simulink library "AERO_lib"  (R2015a)
settings: Solver=ode45  StartTime=0.0  StopTime=10.0  RelTol=1e-3
values from neighbouring files (symbols this model uses):
  AERO = AEROmod    [setup_aero.m]
undefined symbols (not defined in the file or in its folder): VAF
libraries: STRUCT_MDL x2, simulink x2
settings Model: Creator=Andrew  LastModifiedBy=Andrew

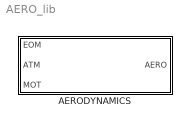
== system AERO_lib ==
  AERODYNAMICS : Subsystem

== system AERO_lib/AERODYNAMICS ==
  EOM : Inport
  ATM : Inport  Port=2
  MOT : Inport  Port=3
  AERODYNAMICS : Subsystem
  Bus Creator : BusCreator  Inputs=3
  Bus Selector : BusSelector  OutputSignals=SONIC_VEL,TEMP,RHO
  Bus Selector1 : BusSelector  OutputSignals=signal1,signal2
  Bus Selector2 : BusSelector  OutputSignals=signal1,signal2
  AERO : Outport
  wires:
  Bus Selector2/2 -> AERODYNAMICS/9(MOTOR DIAMETER)  "<signal2>"
  Bus Selector2/1 -> AERODYNAMICS/8(THRUST ACTIVE)  "<signal1>"
  Bus Selector/3 -> AERODYNAMICS/7(RHO)  "<RHO>"
  Bus Selector/2 -> AERODYNAMICS/6(TEMP)  "<TEMP>"
  Bus Selector/1 -> AERODYNAMICS/5(a (m/s))  "<SONIC_VEL>"
  Bus Creator/1 -> AERO/1
  ATM/1 -> Bus Selector/1
  EOM/1 -> Bus Selector1/1
  MOT/1 -> Bus Selector2/1
  AERODYNAMICS/2(VEHICLE) -> Bus Creator/2  "VEHICLE"
  AERODYNAMICS/3(FLUID) -> Bus Creator/3  "FLUID"
  AERODYNAMICS/1(AERO_PROP) -> Bus Creator/1  "AERO_PROP"

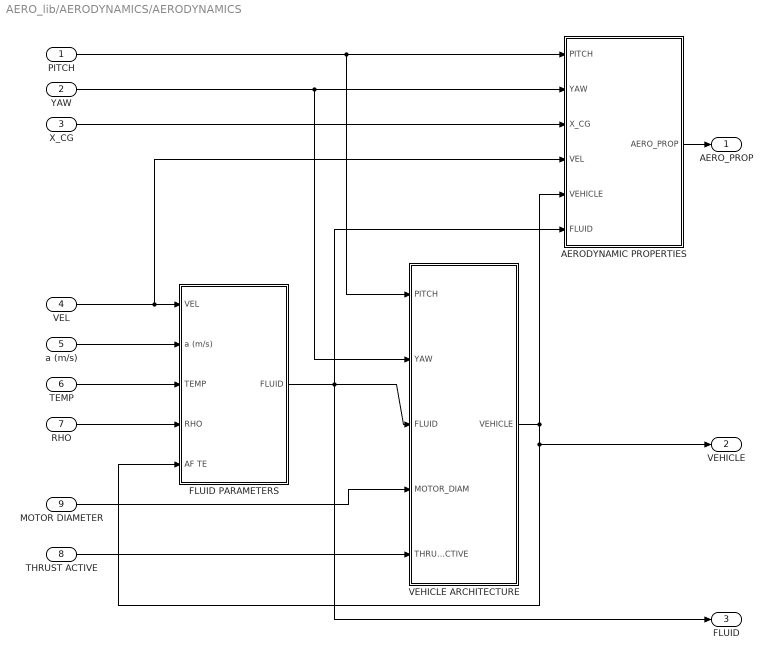
== system AERO_lib/AERODYNAMICS/AERODYNAMICS ==
  PITCH : Inport
  YAW : Inport  Port=2
  X_CG : Inport  Port=3
  VEL : Inport  Port=4
  a (m/s) : Inport  Port=5
  TEMP : Inport  Port=6
  RHO : Inport  Port=7
  THRUST ACTIVE : Inport  Port=8
  MOTOR DIAMETER : Inport  Port=9
  AERODYNAMIC PROPERTIES : Subsystem
  FLUID PARAMETERS : Subsystem
  VEHICLE ARCHITECTURE : Subsystem
  AERO_PROP : Outport
  VEHICLE : Outport  Port=2
  FLUID : Outport  Port=3
  wires:
  TEMP/1 -> FLUID PARAMETERS/3(TEMP)
  THRUST ACTIVE/1 -> VEHICLE ARCHITECTURE/5(THRUST_ACTIVE)
  MOTOR DIAMETER/1 -> VEHICLE ARCHITECTURE/4(MOTOR_DIAM)
  VEHICLE ARCHITECTURE/1(VEHICLE) -> FLUID PARAMETERS/5(AF TE), VEHICLE/1, AERODYNAMIC PROPERTIES/5(VEHICLE)
  RHO/1 -> FLUID PARAMETERS/4(RHO)
  a (m/s)/1 -> FLUID PARAMETERS/2(a (m/s))
  PITCH/1 -> VEHICLE ARCHITECTURE/1(PITCH), AERODYNAMIC PROPERTIES/1(PITCH)
  VEL/1 -> AERODYNAMIC PROPERTIES/4(VEL), FLUID PARAMETERS/1(VEL)
  X_CG/1 -> AERODYNAMIC PROPERTIES/3(X_CG)
  FLUID PARAMETERS/1(FLUID) -> AERODYNAMIC PROPERTIES/6(FLUID), VEHICLE ARCHITECTURE/3(FLUID), FLUID/1
  AERODYNAMIC PROPERTIES/1(AERO_PROP) -> AERO_PROP/1
  YAW/1 -> VEHICLE ARCHITECTURE/2(YAW), AERODYNAMIC PROPERTIES/2(YAW)

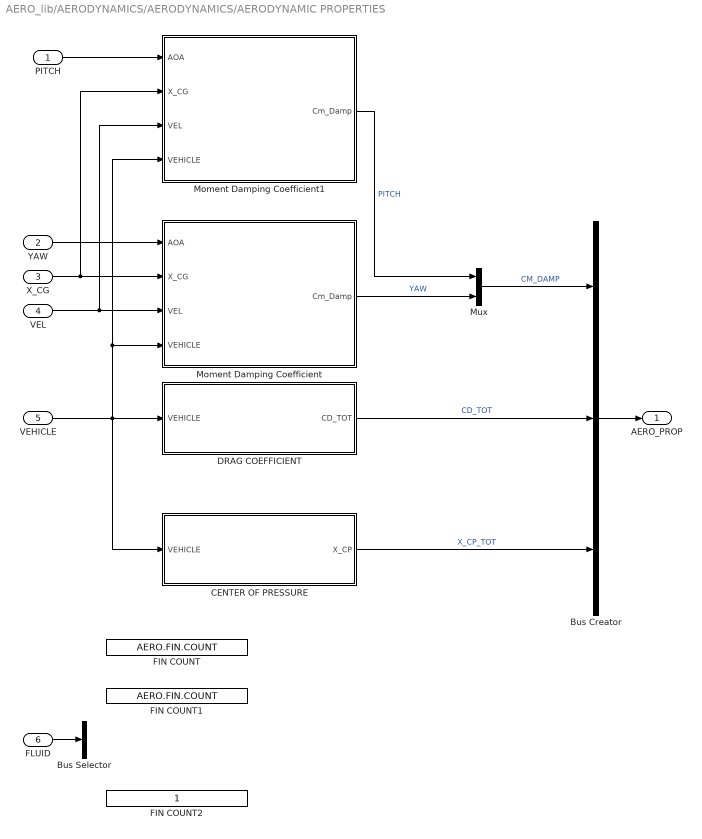
== system AERO_lib/AERODYNAMICS/AERODYNAMICS/AERODYNAMIC PROPERTIES ==
  PITCH : Inport
  YAW : Inport  Port=2
  X_CG : Inport  Port=3
  VEL : Inport  Port=4
  VEHICLE : Inport  Port=5
  FLUID : Inport  Port=6
  Bus Creator : BusCreator  Inputs=3
  Bus Selector : BusSelector  OutputSignals=MACH
  CENTER OF PRESSURE : Subsystem
  DRAG COEFFICIENT : Subsystem
  FIN COUNT : Constant  Value=AERO.FIN.COUNT
  FIN COUNT1 : Constant  Value=AERO.FIN.COUNT
  FIN COUNT2 : Constant
  Moment Damping Coefficient : Subsystem
  Moment Damping Coefficient1 : Subsystem
  Mux : Mux  Inputs=2
  AERO_PROP : Outport
  wires:
  VEL/1 -> Moment Damping Coefficient/3(VEL), Moment Damping Coefficient1/3(VEL)
  X_CG/1 -> Moment Damping Coefficient/2(X_CG), Moment Damping Coefficient1/2(X_CG)
  PITCH/1 -> Moment Damping Coefficient1/1(AOA)
  VEHICLE/1 -> CENTER OF PRESSURE/1(VEHICLE), Moment Damping Coefficient1/4(VEHICLE), Moment Damping Coefficient/4(VEHICLE), DRAG COEFFICIENT/1(VEHICLE)
  DRAG COEFFICIENT/1(CD_TOT) -> Bus Creator/2  "CD_TOT"
  CENTER OF PRESSURE/1(X_CP) -> Bus Creator/3  "X_CP_TOT"
  Bus Creator/1 -> AERO_PROP/1
  YAW/1 -> Moment Damping Coefficient/1(AOA)
  Moment Damping Coefficient/1(Cm_Damp) -> Mux/2  "YAW"
  Moment Damping Coefficient1/1(Cm_Damp) -> Mux/1  "PITCH"
  Mux/1 -> Bus Creator/1  "CM_DAMP"
  FLUID/1 -> Bus Selector/1

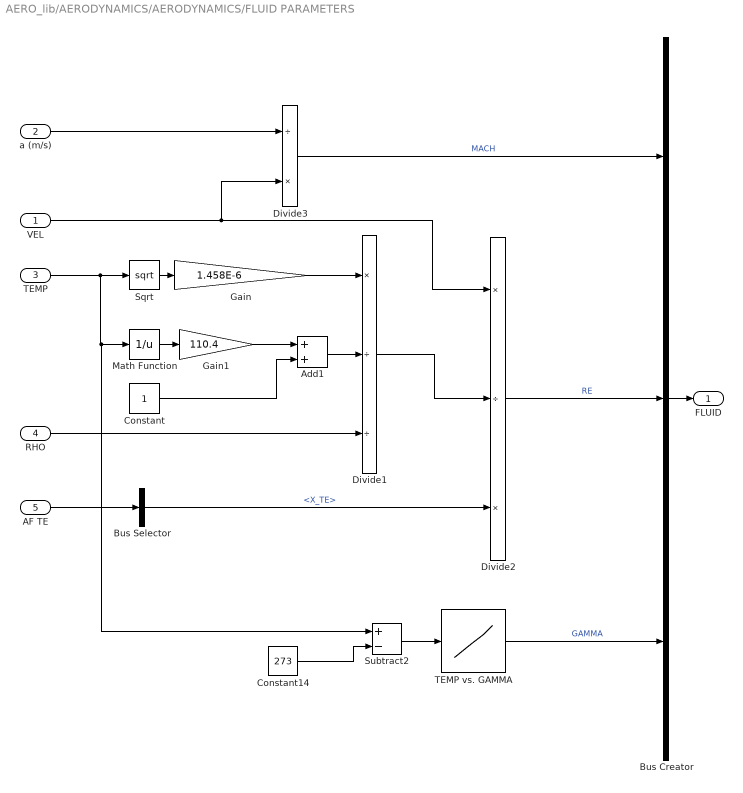
== system AERO_lib/AERODYNAMICS/AERODYNAMICS/FLUID PARAMETERS ==
  VEL : Inport
  a (m/s) : Inport  Port=2
  TEMP : Inport  Port=3
  RHO : Inport  Port=4
  AF TE : Inport  Port=5
  Add1 : Sum
  Bus Creator : BusCreator  Inputs=3
  Bus Selector : BusSelector  OutputSignals=AIRFRAME.AF_2.X_TE
  Constant : Constant
  Constant14 : Constant  Value=273
  Divide1 : Product  Inputs=*//
  Divide2 : Product  Inputs=*/*
  Divide3 : Product  Inputs=/*
  Gain : Gain  Gain=1.458E-6
  Gain1 : Gain  Gain=110.4
  Math Function : Math  Operator=reciprocal  SaturateOnIntegerOverflow=on
  Sqrt : Sqrt  SaturateOnIntegerOverflow=on
  Subtract2 : Sum  Inputs=+-
  TEMP vs. GAMMA : Lookup_n-D  NumberOfTableDimensions=1  BreakpointsForDimension1=VAF.GAS.GAMMA_VS_TEMP(:,1)  Table=VAF.GAS.GAMMA_VS_TEMP(:,2)  InternalRulePriority=Speed  RndMeth=Simplest  InputSameDT=on
  FLUID : Outport
  wires:
  Constant/1 -> Add1/2
  Math Function/1 -> Gain1/1
  Gain1/1 -> Add1/1
  RHO/1 -> Divide1/3
  Add1/1 -> Divide1/2
  Divide1/1 -> Divide2/2
  Sqrt/1 -> Gain/1
  Gain/1 -> Divide1/1
  Divide2/1 -> Bus Creator/2  "RE"
  VEL/1 -> Divide3/2, Divide2/1
  a (m/s)/1 -> Divide3/1
  Divide3/1 -> Bus Creator/1  "MACH"
  Subtract2/1 -> TEMP vs. GAMMA/1
  TEMP/1 -> Subtract2/1, Math Function/1, Sqrt/1
  Constant14/1 -> Subtract2/2
  TEMP vs. GAMMA/1 -> Bus Creator/3  "GAMMA"
  AF TE/1 -> Bus Selector/1
  Bus Selector/1 -> Divide2/3  "<X_TE>"
  Bus Creator/1 -> FLUID/1

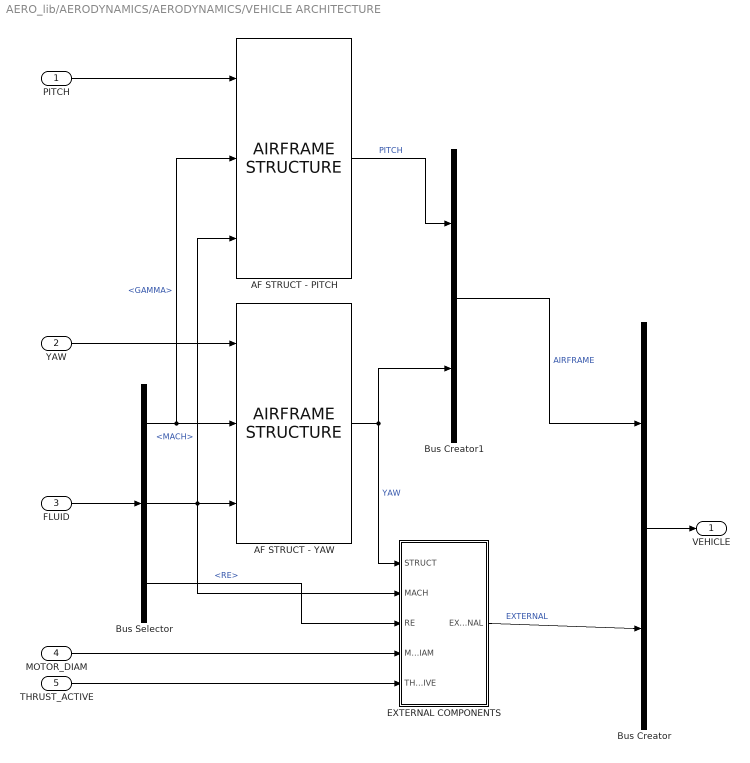
== system AERO_lib/AERODYNAMICS/AERODYNAMICS/VEHICLE ARCHITECTURE ==
  PITCH : Inport
  YAW : Inport  Port=2
  FLUID : Inport  Port=3
  MOTOR_DIAM : Inport  Port=4
  THRUST_ACTIVE : Inport  Port=5
  AF STRUCT - PITCH : STRUCT_MDL/AIRFRAME STRUCTURE
  AF STRUCT - YAW : STRUCT_MDL/AIRFRAME STRUCTURE
  Bus Creator : BusCreator  Inputs=2
  Bus Creator1 : BusCreator  Inputs=2
  Bus Selector : BusSelector  OutputSignals=GAMMA,MACH,RE
  EXTERNAL COMPONENTS : Subsystem
  VEHICLE : Outport
  wires:
  MOTOR_DIAM/1 -> EXTERNAL COMPONENTS/4(MOTOR_DIAM)
  THRUST_ACTIVE/1 -> EXTERNAL COMPONENTS/5(THRUST_ACTIVE)
  AF STRUCT - YAW/1 -> EXTERNAL COMPONENTS/1(STRUCT), Bus Creator1/2  "YAW"
  EXTERNAL COMPONENTS/1(EXTERNAL) -> Bus Creator/2  "EXTERNAL"
  Bus Creator/1 -> VEHICLE/1
  FLUID/1 -> Bus Selector/1
  Bus Selector/1 -> AF STRUCT - PITCH/2, AF STRUCT - YAW/2  "<GAMMA>"
  Bus Selector/3 -> EXTERNAL COMPONENTS/3(RE)  "<RE>"
  Bus Selector/2 -> AF STRUCT - PITCH/3, AF STRUCT - YAW/3, EXTERNAL COMPONENTS/2(MACH)  "<MACH>"
  PITCH/1 -> AF STRUCT - PITCH/1
  YAW/1 -> AF STRUCT - YAW/1
  Bus Creator1/1 -> Bus Creator/1  "AIRFRAME"
  AF STRUCT - PITCH/1 -> Bus Creator1/1  "PITCH"

== system AERO_lib/AERODYNAMICS/AERODYNAMICS/AERODYNAMIC PROPERTIES/CENTER OF PRESSURE ==
  VEHICLE : Inport
  Bus Selector : BusSelector  OutputSignals=NC.CP,AF_1.CP,AF_2.CP,FIN.CP,NC.CN_ALPHA,AF_1.CN_ALPHA,AF_2.CN_ALPHA,FIN.CN_ALPHA
  Divide : Product  Inputs=*/
  Dot Product : DotProduct  InputSameDT=on  OutDataTypeStr=Inherit: Inherit via internal rule
  Mux : Mux
  Mux1 : Mux
  Sum of Elements1 : Sum  Inputs=+
  X_CP : Outport
  wires:
  Divide/1 -> X_CP/1  "X_CP_TOT"
  VEHICLE/1 -> Bus Selector/1
  Mux1/1 -> Dot Product/2, Sum of Elements1/1
  Sum of Elements1/1 -> Divide/2
  Mux/1 -> Dot Product/1
  Bus Selector/4 -> Mux/4  "<CP>"
  Bus Selector/3 -> Mux/3  "<CP>"
  Bus Selector/2 -> Mux/2  "<CP>"
  Bus Selector/1 -> Mux/1  "<CP>"
  Bus Selector/5 -> Mux1/1  "<CN_ALPHA>"
  Bus Selector/6 -> Mux1/2  "<CN_ALPHA>"
  Bus Selector/7 -> Mux1/3  "<CN_ALPHA>"
  Bus Selector/8 -> Mux1/4  "<CN_ALPHA>"
  Dot Product/1 -> Divide/1

== system AERO_lib/AERODYNAMICS/AERODYNAMICS/AERODYNAMIC PROPERTIES/DRAG COEFFICIENT ==
  VEHICLE : Inport
  Add1 : Sum
  Bus Selector1 : BusSelector  OutputSignals=EXTERNAL.SKIN_EFFECTS,AIRFRAME.NC.CD,AIRFRAME.FIN.CD,EXTERNAL.BASE.CD_BASE,EXTERNAL.PARASITIC.CD_PARASITIC,AIRFRAME.NC.REF_AREA,AIRFRAME.FIN.REF_AREA,EXTERNAL.BASE.BASE_REF_AREA,EXTERNAL.PARASITIC.AREA_PARASITIC,AIRFRAME.AF_1.AREA_LE
  Divide1 : Product  Inputs=*/
  Dot Product1 : DotProduct  InputSameDT=on  OutDataTypeStr=Inherit: Inherit via internal rule
  Mux3 : Mux
  Mux4 : Mux
  CD_TOT : Outport
  wires:
  Mux3/1 -> Dot Product1/1
  VEHICLE/1 -> Bus Selector1/1
  Mux4/1 -> Dot Product1/2
  Dot Product1/1 -> Divide1/1
  Bus Selector1/7 -> Mux4/2  "<REF_AREA>"
  Bus Selector1/8 -> Mux4/3  "<BASE_REF_AREA>"
  Bus Selector1/9 -> Mux4/4  "<AREA_PARASITIC>"
  Bus Selector1/2 -> Mux3/1  "<CD>"
  Bus Selector1/1 -> Add1/1  "<SKIN_EFFECTS>"
  Divide1/1 -> Add1/2
  Add1/1 -> CD_TOT/1  "CD_TOT"
  Bus Selector1/6 -> Mux4/1  "<REF_AREA>"
  Bus Selector1/4 -> Mux3/3  "<CD_BASE>"
  Bus Selector1/3 -> Mux3/2  "<CD>"
  Bus Selector1/5 -> Mux3/4  "<CD_PARASITIC>"
  Bus Selector1/10 -> Divide1/2  "<AREA_LE>"

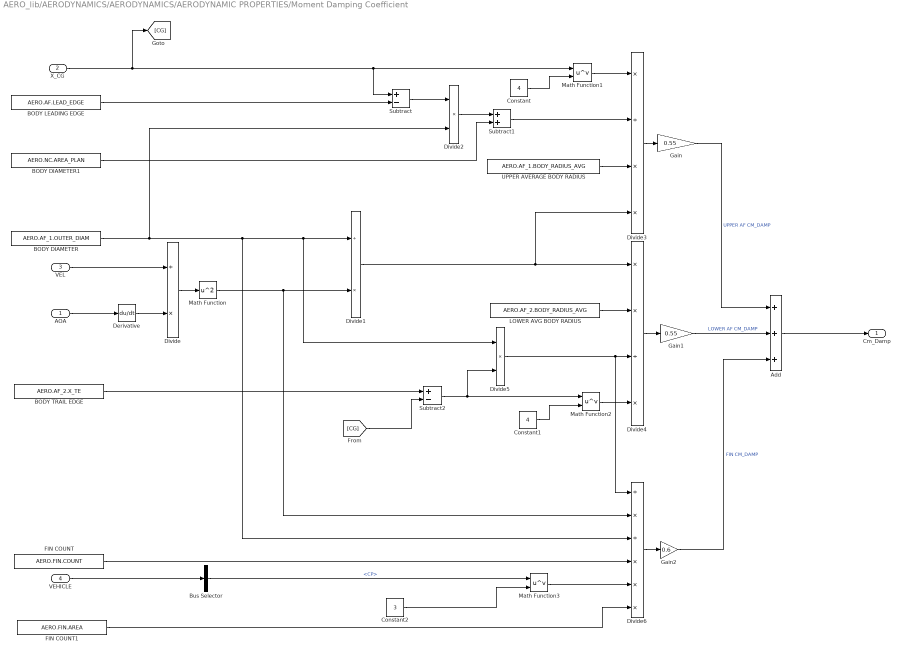
== system AERO_lib/AERODYNAMICS/AERODYNAMICS/AERODYNAMIC PROPERTIES/Moment Damping Coefficient ==
  AOA : Inport
  X_CG : Inport  Port=2
  VEL : Inport  Port=3
  VEHICLE : Inport  Port=4
  Add : Sum  Inputs=+++
  BODY DIAMETER : FromWorkspace  VariableName=AERO.AF_1.OUTER_DIAM  SampleTime=0
  BODY DIAMETER1 : FromWorkspace  VariableName=AERO.NC.AREA_PLAN  SampleTime=0
  BODY LEADING EDGE : FromWorkspace  VariableName=AERO.AF.LEAD_EDGE  SampleTime=0
  BODY TRAIL EDGE : Constant  Value=AERO.AF_2.X_TE
  Bus Selector : BusSelector  OutputSignals=AIRFRAME.YAW.FIN.CP
  Constant : Constant  Value=4
  Constant1 : Constant  Value=4
  Constant2 : Constant  Value=3
  Derivative : Derivative
  Divide : Product  Inputs=/*
  Divide1 : Product  Inputs=/*
  Divide2 : Product  Inputs=**
  Divide3 : Product  Inputs=*/**
  Divide4 : Product  Inputs=**/*
  Divide5 : Product  Inputs=**
  Divide6 : Product  Inputs=/*/***
  FIN COUNT : Constant  Value=AERO.FIN.COUNT
  FIN COUNT1 : FromWorkspace  VariableName=AERO.FIN.AREA  SampleTime=0
  Gain : Gain  Gain=0.55
  Gain1 : Gain  Gain=0.55
  Gain2 : Gain  Gain=0.6
  LOWER AVG BODY RADIUS : FromWorkspace  VariableName=AERO.AF_2.BODY_RADIUS_AVG  SampleTime=0
  Math Function : Math  Operator=square  SaturateOnIntegerOverflow=on
  Math Function1 : Math  Operator=pow  SaturateOnIntegerOverflow=on
  Math Function2 : Math  Operator=pow  SaturateOnIntegerOverflow=on
  Math Function3 : Math  Operator=pow  SaturateOnIntegerOverflow=on
  Subtract : Sum  Inputs=+-
  Subtract1 : Sum
  Subtract2 : Sum  Inputs=+-
  UPPER AVERAGE BODY RADIUS : Constant  Value=AERO.AF_1.BODY_RADIUS_AVG
  Cm_Damp : Outport
  wires:
  Derivative/1 -> Divide/2
  VEL/1 -> Divide/1
  Divide/1 -> Math Function/1
  Math Function/1 -> Divide6/2, Divide1/2
  BODY LEADING EDGE/1 -> Subtract/2
  Divide2/1 -> Subtract1/1
  Constant/1 -> Math Function1/2
  Subtract/1 -> Divide2/1
  Subtract1/1 -> Divide3/2
  BODY DIAMETER1/1 -> Subtract1/2
  BODY DIAMETER/1 -> Divide6/3, Divide5/1, Divide1/1, Divide2/2
  X_CG/1 -> [CG], Subtract/1, Math Function1/1
  Math Function1/1 -> Divide3/1
  Divide3/1 -> Gain/1
  BODY TRAIL EDGE/1 -> Subtract2/1
  [CG] -> Subtract2/2
  Divide5/1 -> Divide6/1, Divide4/3
  Subtract2/1 -> Math Function2/1, Divide5/2
  Constant1/1 -> Math Function2/2
  Divide4/1 -> Gain1/1
  VEHICLE/1 -> Bus Selector/1
  Constant2/1 -> Math Function3/2
  Math Function3/1 -> Divide6/5
  FIN COUNT/1 -> Divide6/4
  FIN COUNT1/1 -> Divide6/6
  Divide6/1 -> Gain2/1
  Gain1/1 -> Add/2  "LOWER AF CM_DAMP"
  Gain2/1 -> Add/3  "FIN CM_DAMP"
  Gain/1 -> Add/1  "UPPER AF CM_DAMP"
  UPPER AVERAGE BODY RADIUS/1 -> Divide3/3
  Divide1/1 -> Divide3/4, Divide4/1
  Math Function2/1 -> Divide4/4
  LOWER AVG BODY RADIUS/1 -> Divide4/2
  Bus Selector/1 -> Math Function3/1  "<CP>"
  AOA/1 -> Derivative/1
  Add/1 -> Cm_Damp/1

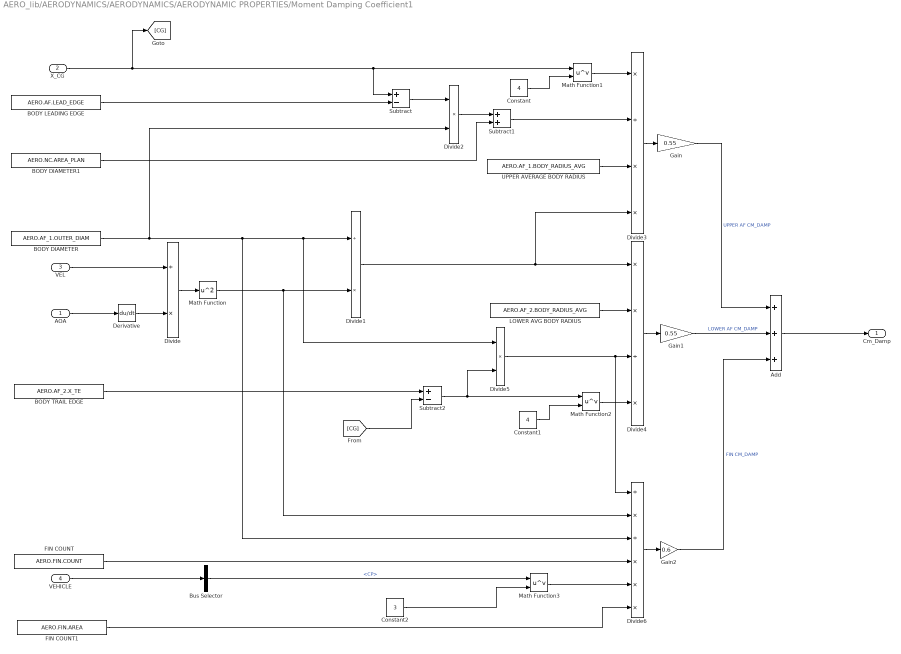
== system AERO_lib/AERODYNAMICS/AERODYNAMICS/AERODYNAMIC PROPERTIES/Moment Damping Coefficient1 ==
  AOA : Inport
  X_CG : Inport  Port=2
  VEL : Inport  Port=3
  VEHICLE : Inport  Port=4
  Add : Sum  Inputs=+++
  BODY DIAMETER : FromWorkspace  VariableName=AERO.AF_1.OUTER_DIAM  SampleTime=0
  BODY DIAMETER1 : FromWorkspace  VariableName=AERO.NC.AREA_PLAN  SampleTime=0
  BODY LEADING EDGE : FromWorkspace  VariableName=AERO.AF.LEAD_EDGE  SampleTime=0
  BODY TRAIL EDGE : Constant  Value=AERO.AF_2.X_TE
  Bus Selector : BusSelector  OutputSignals=AIRFRAME.PITCH.FIN.CP
  Constant : Constant  Value=4
  Constant1 : Constant  Value=4
  Constant2 : Constant  Value=3
  Derivative : Derivative
  Divide : Product  Inputs=/*
  Divide1 : Product  Inputs=/*
  Divide2 : Product  Inputs=**
  Divide3 : Product  Inputs=*/**
  Divide4 : Product  Inputs=**/*
  Divide5 : Product  Inputs=**
  Divide6 : Product  Inputs=/*/***
  FIN COUNT : Constant  Value=AERO.FIN.COUNT
  FIN COUNT1 : FromWorkspace  VariableName=AERO.FIN.AREA  SampleTime=0
  Gain : Gain  Gain=0.55
  Gain1 : Gain  Gain=0.55
  Gain2 : Gain  Gain=0.6
  LOWER AVG BODY RADIUS : FromWorkspace  VariableName=AERO.AF_2.BODY_RADIUS_AVG  SampleTime=0
  Math Function : Math  Operator=square  SaturateOnIntegerOverflow=on
  Math Function1 : Math  Operator=pow  SaturateOnIntegerOverflow=on
  Math Function2 : Math  Operator=pow  SaturateOnIntegerOverflow=on
  Math Function3 : Math  Operator=pow  SaturateOnIntegerOverflow=on
  Subtract : Sum  Inputs=+-
  Subtract1 : Sum
  Subtract2 : Sum  Inputs=+-
  UPPER AVERAGE BODY RADIUS : Constant  Value=AERO.AF_1.BODY_RADIUS_AVG
  Cm_Damp : Outport
  wires:
  Add/1 -> Cm_Damp/1
  AOA/1 -> Derivative/1
  Bus Selector/1 -> Math Function3/1  "<CP>"
  LOWER AVG BODY RADIUS/1 -> Divide4/2
  Math Function2/1 -> Divide4/4
  Divide1/1 -> Divide4/1, Divide3/4
  UPPER AVERAGE BODY RADIUS/1 -> Divide3/3
  Gain/1 -> Add/1  "UPPER AF CM_DAMP"
  Gain2/1 -> Add/3  "FIN CM_DAMP"
  Gain1/1 -> Add/2  "LOWER AF CM_DAMP"
  Divide6/1 -> Gain2/1
  FIN COUNT1/1 -> Divide6/6
  FIN COUNT/1 -> Divide6/4
  Math Function3/1 -> Divide6/5
  Constant2/1 -> Math Function3/2
  VEHICLE/1 -> Bus Selector/1
  Divide4/1 -> Gain1/1
  Constant1/1 -> Math Function2/2
  Subtract2/1 -> Divide5/2, Math Function2/1
  Divide5/1 -> Divide4/3, Divide6/1
  [CG] -> Subtract2/2
  BODY TRAIL EDGE/1 -> Subtract2/1
  Divide3/1 -> Gain/1
  Math Function1/1 -> Divide3/1
  X_CG/1 -> Math Function1/1, Subtract/1, [CG]
  BODY DIAMETER/1 -> Divide2/2, Divide1/1, Divide5/1, Divide6/3
  BODY DIAMETER1/1 -> Subtract1/2
  Subtract1/1 -> Divide3/2
  Subtract/1 -> Divide2/1
  Constant/1 -> Math Function1/2
  Divide2/1 -> Subtract1/1
  BODY LEADING EDGE/1 -> Subtract/2
  Math Function/1 -> Divide1/2, Divide6/2
  Divide/1 -> Math Function/1
  VEL/1 -> Divide/1
  Derivative/1 -> Divide/2

== system AERO_lib/AERODYNAMICS/AERODYNAMICS/VEHICLE ARCHITECTURE/EXTERNAL COMPONENTS ==
  STRUCT : Inport
  MACH : Inport  Port=2
  RE : Inport  Port=3
  MOTOR_DIAM : Inport  Port=4
  THRUST_ACTIVE : Inport  Port=5
  BASE : Subsystem
  Bus Creator : BusCreator  Inputs=3
  Bus Selector : BusSelector  OutputSignals=AF_2.AREA_TE
  PARASITIC : Subsystem
  Skin Friction Drag : Subsystem
  EXTERNAL : Outport
  wires:
  THRUST_ACTIVE/1 -> BASE/3(THRUST ACTIVE)
  MOTOR_DIAM/1 -> BASE/2(MOTOR DIAMETER)
  RE/1 -> Skin Friction Drag/1(Re)
  BASE/1(BASE) -> Bus Creator/1  "BASE"
  Skin Friction Drag/1(Cd_Fric) -> Bus Creator/3  "SKIN_EFFECTS"
  Bus Creator/1 -> EXTERNAL/1
  MACH/1 -> Skin Friction Drag/2(MACH), PARASITIC/1(MACH), BASE/1(MACH)
  STRUCT/1 -> Bus Selector/1
  Bus Selector/1 -> BASE/4(AF TE AREA)  "<AREA_TE>"
  PARASITIC/1(PARASITIC) -> Bus Creator/2  "PARASITIC"

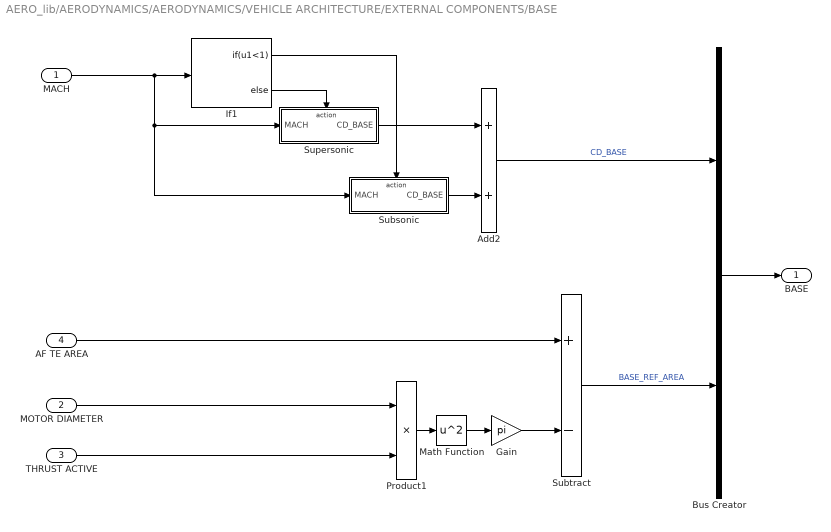
== system AERO_lib/AERODYNAMICS/AERODYNAMICS/VEHICLE ARCHITECTURE/EXTERNAL COMPONENTS/BASE ==
  MACH : Inport
  MOTOR DIAMETER : Inport  Port=2
  THRUST ACTIVE : Inport  Port=3
  AF TE AREA : Inport  Port=4
  Add2 : Sum
  Bus Creator : BusCreator  Inputs=2
  Gain : Gain  Gain=pi
  If1 : If  IfExpression=u1<1
  Math Function : Math  Operator=square  SaturateOnIntegerOverflow=on
  Product1 : Product
  Subsonic : Subsystem  TreatAsAtomicUnit=on
  Subtract : Sum  Inputs=+-
  Supersonic : Subsystem  TreatAsAtomicUnit=on
  BASE : Outport
  wires:
  Add2/1 -> Bus Creator/1  "CD_BASE"
  Subtract/1 -> Bus Creator/2  "BASE_REF_AREA"
  AF TE AREA/1 -> Subtract/1
  Product1/1 -> Math Function/1
  THRUST ACTIVE/1 -> Product1/2
  MOTOR DIAMETER/1 -> Product1/1
  Gain/1 -> Subtract/2
  Math Function/1 -> Gain/1
  If1/2 -> Supersonic/Action
  If1/1 -> Subsonic/Action
  Subsonic/1(CD_BASE) -> Add2/2
  Supersonic/1(CD_BASE) -> Add2/1
  MACH/1 -> Subsonic/1(MACH), Supersonic/1(MACH), If1/1
  Bus Creator/1 -> BASE/1

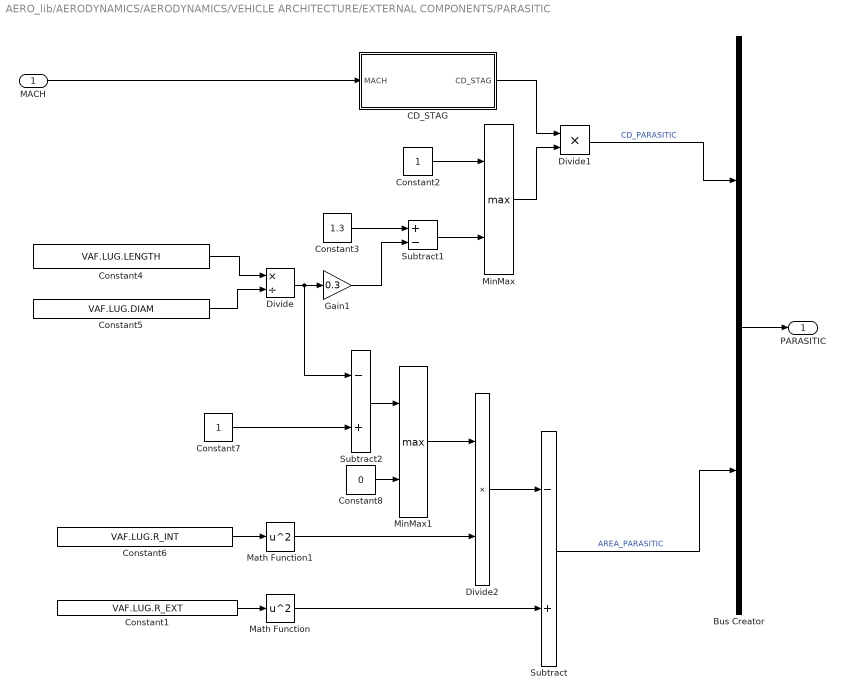
== system AERO_lib/AERODYNAMICS/AERODYNAMICS/VEHICLE ARCHITECTURE/EXTERNAL COMPONENTS/PARASITIC ==
  MACH : Inport
  Bus Creator : BusCreator  Inputs=2
  CD_STAG : Subsystem
  Constant1 : Constant  Value=VAF.LUG.R_EXT
  Constant2 : Constant
  Constant3 : Constant  Value=1.3
  Constant4 : Constant  Value=VAF.LUG.LENGTH
  Constant5 : Constant  Value=VAF.LUG.DIAM
  Constant6 : Constant  Value=VAF.LUG.R_INT
  Constant7 : Constant
  Constant8 : Constant  Value=0
  Divide : Product  Inputs=*/
  Divide1 : Product  Inputs=**
  Divide2 : Product  Inputs=**
  Gain1 : Gain  Gain=0.3
  Math Function : Math  Operator=square  SaturateOnIntegerOverflow=on
  Math Function1 : Math  Operator=square  SaturateOnIntegerOverflow=on
  MinMax : MinMax  Function=max  Inputs=2
  MinMax1 : MinMax  Function=max  Inputs=2
  Subtract : Sum  Inputs=-+
  Subtract1 : Sum  Inputs=+-
  Subtract2 : Sum  Inputs=-+
  PARASITIC : Outport
  wires:
  Divide1/1 -> Bus Creator/1  "CD_PARASITIC"
  Subtract1/1 -> MinMax/2
  Constant3/1 -> Subtract1/1
  Gain1/1 -> Subtract1/2
  Constant2/1 -> MinMax/1
  Divide/1 -> Subtract2/1, Gain1/1
  Constant5/1 -> Divide/2
  Constant4/1 -> Divide/1
  CD_STAG/1(CD_STAG) -> Divide1/1
  MinMax/1 -> Divide1/2
  MACH/1 -> CD_STAG/1(MACH)
  Constant1/1 -> Math Function/1
  Math Function/1 -> Subtract/2
  Constant6/1 -> Math Function1/1
  Constant7/1 -> Subtract2/2
  Subtract2/1 -> MinMax1/1
  Constant8/1 -> MinMax1/2
  MinMax1/1 -> Divide2/1
  Math Function1/1 -> Divide2/2
  Divide2/1 -> Subtract/1
  Subtract/1 -> Bus Creator/2  "AREA_PARASITIC"
  Bus Creator/1 -> PARASITIC/1

== system AERO_lib/AERODYNAMICS/AERODYNAMICS/VEHICLE ARCHITECTURE/EXTERNAL COMPONENTS/Skin Friction Drag ==
  Re : Inport
  MACH : Inport  Port=2
  Compressibility Corrections : Subsystem
  Friction Drag Coefficient : Subsystem
  RE-BASED FRIC. COEFF : Subsystem
  Cd_Fric : Outport
  wires:
  Re/1 -> RE-BASED FRIC. COEFF/1(RE)
  RE-BASED FRIC. COEFF/1(CF_Skin) -> Compressibility Corrections/1(RE)
  MACH/1 -> Compressibility Corrections/2(CF_skin)
  Compressibility Corrections/1(CF_Skin) -> Friction Drag Coefficient/1(CF_Skin)
  Friction Drag Coefficient/1(Cd_Fric) -> Cd_Fric/1

== system AERO_lib/AERODYNAMICS/AERODYNAMICS/VEHICLE ARCHITECTURE/EXTERNAL COMPONENTS/BASE/Subsonic ==
  note: CD_LE = 1 + M^2/4 + M^4 / 40
  MACH : Inport
  Action Port : ActionPort
  Constant : Constant  Value=0.12
  Gain : Gain  Gain=0.13
  Math Function : Math  Operator=square  SaturateOnIntegerOverflow=on
  Subtract : Sum
  CD_BASE : Outport
  wires:
  Constant/1 -> Subtract/2
  Math Function/1 -> Gain/1
  MACH/1 -> Math Function/1
  Subtract/1 -> CD_BASE/1
  Gain/1 -> Subtract/1

== system AERO_lib/AERODYNAMICS/AERODYNAMICS/VEHICLE ARCHITECTURE/EXTERNAL COMPONENTS/BASE/Supersonic ==
  MACH : Inport
  Action Port : ActionPort
  Gain : Gain  Gain=0.25
  Math Function : Math  Operator=reciprocal  SaturateOnIntegerOverflow=on
  CD_BASE : Outport
  wires:
  Gain/1 -> CD_BASE/1
  MACH/1 -> Math Function/1
  Math Function/1 -> Gain/1

== system AERO_lib/AERODYNAMICS/AERODYNAMICS/VEHICLE ARCHITECTURE/EXTERNAL COMPONENTS/PARASITIC/CD_STAG ==
  MACH : Inport
  Add1 : Sum
  If : If  IfExpression=u1<1
  Subsonic : Subsystem  TreatAsAtomicUnit=on
  Supersonic : Subsystem  TreatAsAtomicUnit=on
  CD_STAG : Outport
  wires:
  MACH/1 -> If/1, Subsonic/1(MACH), Supersonic/1(MACH)
  Supersonic/1(CD_STAG) -> Add1/1
  Subsonic/1(CD_STAG) -> Add1/2
  If/1 -> Subsonic/Action
  If/2 -> Supersonic/Action
  Add1/1 -> CD_STAG/1

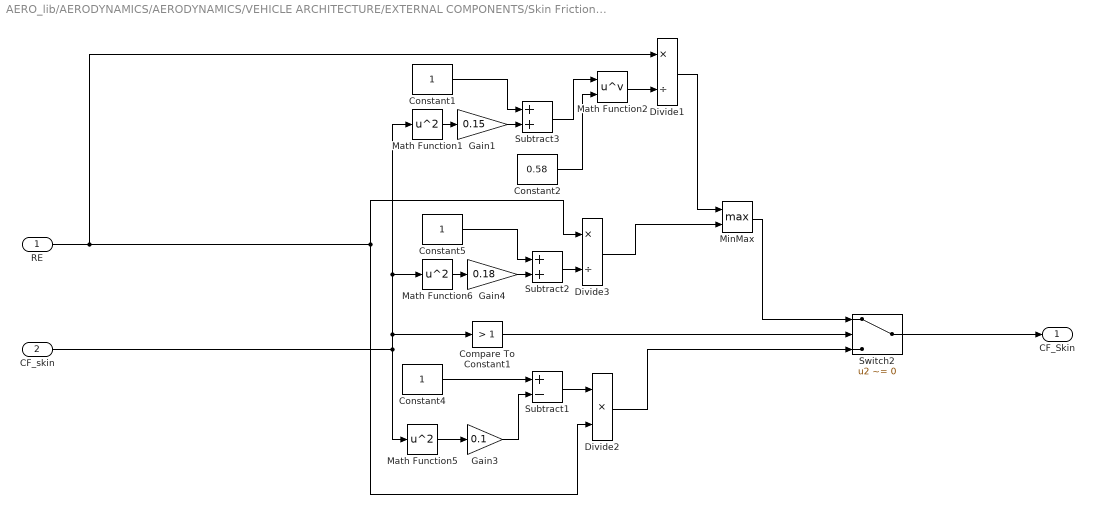
== system AERO_lib/AERODYNAMICS/AERODYNAMICS/VEHICLE ARCHITECTURE/EXTERNAL COMPONENTS/Skin Friction Drag/Compressibility Corrections ==
  RE : Inport
  CF_skin : Inport  Port=2
  Compare To Constant1 : simulink/Logic and Bit Operations/Compare To Constant  relop=>  const=1  OutDataTypeStr=boolean
  Constant1 : Constant
  Constant2 : Constant  Value=0.58
  Constant4 : Constant
  Constant5 : Constant
  Divide1 : Product  Inputs=*/
  Divide2 : Product  Inputs=**
  Divide3 : Product  Inputs=*/
  Gain1 : Gain  Gain=0.15
  Gain3 : Gain  Gain=0.1
  Gain4 : Gain  Gain=0.18
  Math Function1 : Math  Operator=square  SaturateOnIntegerOverflow=on
  Math Function2 : Math  Operator=pow  SaturateOnIntegerOverflow=on
  Math Function5 : Math  Operator=square  SaturateOnIntegerOverflow=on
  Math Function6 : Math  Operator=square  SaturateOnIntegerOverflow=on
  MinMax : MinMax  Function=max  Inputs=2
  Subtract1 : Sum  Inputs=+-
  Subtract2 : Sum
  Subtract3 : Sum
  Switch2 : Switch  Criteria=u2 ~= 0
  CF_Skin : Outport
  wires:
  Subtract1/1 -> Divide2/1
  Math Function2/1 -> Divide1/2
  Constant2/1 -> Math Function2/2
  Subtract3/1 -> Math Function2/1
  Math Function5/1 -> Gain3/1
  Gain3/1 -> Subtract1/2
  Constant4/1 -> Subtract1/1
  Divide2/1 -> Switch2/3
  Compare To Constant1/1 -> Switch2/2
  CF_skin/1 -> Math Function5/1, Math Function1/1, Math Function6/1, Compare To Constant1/1
  Constant1/1 -> Subtract3/1
  Gain1/1 -> Subtract3/2
  Math Function1/1 -> Gain1/1
  Math Function6/1 -> Gain4/1
  Gain4/1 -> Subtract2/2
  MinMax/1 -> Switch2/1
  RE/1 -> Divide1/1, Divide2/2, Divide3/1
  Subtract2/1 -> Divide3/2
  Divide3/1 -> MinMax/2
  Switch2/1 -> CF_Skin/1
  Constant5/1 -> Subtract2/1
  Divide1/1 -> MinMax/1

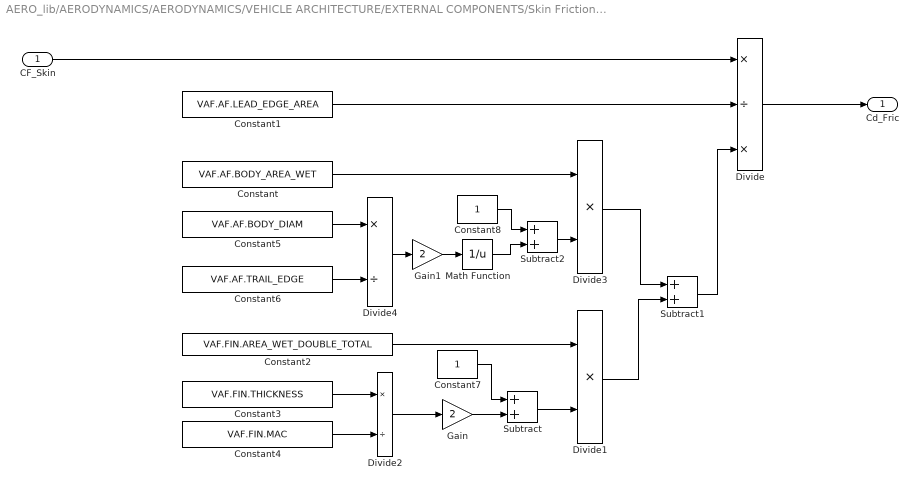
== system AERO_lib/AERODYNAMICS/AERODYNAMICS/VEHICLE ARCHITECTURE/EXTERNAL COMPONENTS/Skin Friction Drag/Friction Drag Coefficient ==
  CF_Skin : Inport
  Constant : Constant  Value=VAF.AF.BODY_AREA_WET
  Constant1 : Constant  Value=VAF.AF.LEAD_EDGE_AREA
  Constant2 : Constant  Value=VAF.FIN.AREA_WET_DOUBLE_TOTAL
  Constant3 : Constant  Value=VAF.FIN.THICKNESS
  Constant4 : Constant  Value=VAF.FIN.MAC
  Constant5 : Constant  Value=VAF.AF.BODY_DIAM
  Constant6 : Constant  Value=VAF.AF.TRAIL_EDGE
  Constant7 : Constant
  Constant8 : Constant
  Divide : Product  Inputs=*/*
  Divide1 : Product  Inputs=**
  Divide2 : Product  Inputs=*/
  Divide3 : Product  Inputs=**
  Divide4 : Product  Inputs=*/
  Gain : Gain  Gain=2
  Gain1 : Gain  Gain=2
  Math Function : Math  Operator=reciprocal  SaturateOnIntegerOverflow=on
  Subtract : Sum
  Subtract1 : Sum
  Subtract2 : Sum
  Cd_Fric : Outport
  wires:
  Gain1/1 -> Math Function/1
  Divide/1 -> Cd_Fric/1
  Divide4/1 -> Gain1/1
  Gain/1 -> Subtract/2
  Constant7/1 -> Subtract/1
  Constant/1 -> Divide3/1
  CF_Skin/1 -> Divide/1
  Subtract2/1 -> Divide3/2
  Constant8/1 -> Subtract2/1
  Math Function/1 -> Subtract2/2
  Subtract1/1 -> Divide/3
  Divide1/1 -> Subtract1/2
  Divide3/1 -> Subtract1/1
  Constant2/1 -> Divide1/1
  Constant6/1 -> Divide4/2
  Constant5/1 -> Divide4/1
  Divide2/1 -> Gain/1
  Constant1/1 -> Divide/2
  Subtract/1 -> Divide1/2
  Constant4/1 -> Divide2/2
  Constant3/1 -> Divide2/1

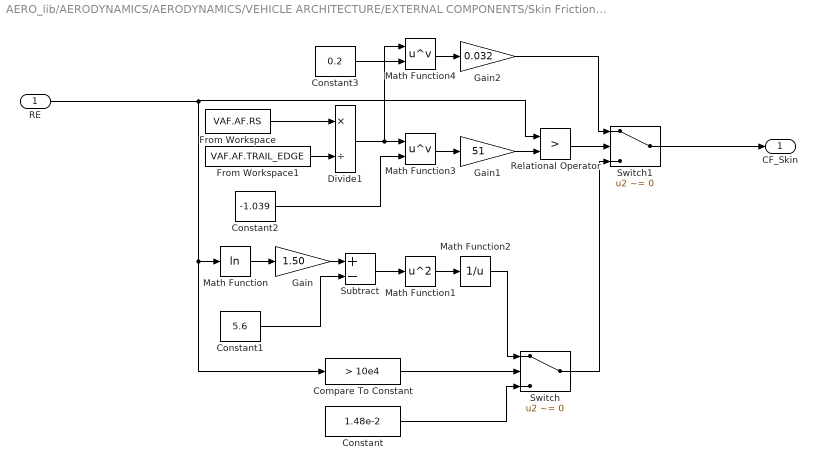
== system AERO_lib/AERODYNAMICS/AERODYNAMICS/VEHICLE ARCHITECTURE/EXTERNAL COMPONENTS/Skin Friction Drag/RE-BASED FRIC. COEFF ==
  RE : Inport
  Compare To Constant : simulink/Logic and Bit Operations/Compare To Constant  relop=>  const=10e4  OutDataTypeStr=boolean
  Constant : Constant  Value=1.48e-2
  Constant1 : Constant  Value=5.6
  Constant2 : Constant  Value=-1.039
  Constant3 : Constant  Value=0.2
  Divide1 : Product  Inputs=*/
  From Workspace : FromWorkspace  VariableName=VAF.AF.RS  SampleTime=0
  From Workspace1 : FromWorkspace  VariableName=VAF.AF.TRAIL_EDGE  SampleTime=0
  Gain : Gain  Gain=1.50
  Gain1 : Gain  Gain=51
  Gain2 : Gain  Gain=0.032
  Math Function : Math  Operator=log  SaturateOnIntegerOverflow=on
  Math Function1 : Math  Operator=square  SaturateOnIntegerOverflow=on
  Math Function2 : Math  Operator=reciprocal  SaturateOnIntegerOverflow=on
  Math Function3 : Math  Operator=pow  SaturateOnIntegerOverflow=on
  Math Function4 : Math  Operator=pow  SaturateOnIntegerOverflow=on
  Relational Operator : RelationalOperator  Operator=>  OutDataTypeStr=boolean
  Subtract : Sum  Inputs=+-
  Switch : Switch  Criteria=u2 ~= 0
  Switch1 : Switch  Criteria=u2 ~= 0
  CF_Skin : Outport
  wires:
  Switch1/1 -> CF_Skin/1
  Compare To Constant/1 -> Switch/2
  From Workspace/1 -> Divide1/1
  From Workspace1/1 -> Divide1/2
  Subtract/1 -> Math Function1/1
  Math Function2/1 -> Switch/1
  Math Function1/1 -> Math Function2/1
  Constant3/1 -> Math Function4/2
  Math Function4/1 -> Gain2/1
  Gain2/1 -> Switch1/1
  Math Function/1 -> Gain/1
  Switch/1 -> Switch1/3
  Constant/1 -> Switch/3
  Relational Operator/1 -> Switch1/2
  Gain1/1 -> Relational Operator/2
  Constant2/1 -> Math Function3/2
  Divide1/1 -> Math Function4/1, Math Function3/1
  Math Function3/1 -> Gain1/1
  RE/1 -> Math Function/1, Compare To Constant/1, Relational Operator/1
  Constant1/1 -> Subtract/2
  Gain/1 -> Subtract/1

== system AERO_lib/AERODYNAMICS/AERODYNAMICS/VEHICLE ARCHITECTURE/EXTERNAL COMPONENTS/PARASITIC/CD_STAG/Subsonic ==
  note: CD_LE = 1 + M^2/4 + M^4 / 40
  MACH : Inport
  Action Port : ActionPort
  Constant : Constant
  Gain : Gain  Gain=0.25
  Gain1 : Gain  Gain=1/40
  Math Function : Math  Operator=square  SaturateOnIntegerOverflow=on
  Math Function1 : Math  Operator=square  SaturateOnIntegerOverflow=on
  Subtract : Sum  Inputs=+++
  CD_STAG : Outport
  wires:
  Math Function/1 -> Gain/1, Math Function1/1
  MACH/1 -> Math Function/1
  Subtract/1 -> CD_STAG/1
  Gain/1 -> Subtract/1
  Math Function1/1 -> Gain1/1
  Gain1/1 -> Subtract/2
  Constant/1 -> Subtract/3

== system AERO_lib/AERODYNAMICS/AERODYNAMICS/VEHICLE ARCHITECTURE/EXTERNAL COMPONENTS/PARASITIC/CD_STAG/Supersonic ==
  MACH : Inport
  Action Port : ActionPort
  Add : Sum  Inputs=+-++
  Constant : Constant  Value=1.84
  Gain : Gain  Gain=0.76
  Gain1 : Gain  Gain=0.166
  Gain2 : Gain  Gain=0.035
  Math Function : Math  Operator=reciprocal  SaturateOnIntegerOverflow=on
  Math Function1 : Math  Operator=square  SaturateOnIntegerOverflow=on
  Math Function2 : Math  Operator=square  SaturateOnIntegerOverflow=on
  Product : Product
  CD_STAG : Outport
  wires:
  Gain/1 -> Add/2
  Constant/1 -> Add/1
  Add/1 -> CD_STAG/1
  MACH/1 -> Math Function/1
  Math Function/1 -> Math Function1/1
  Math Function2/1 -> Gain1/1, Product/1
  Math Function1/1 -> Math Function2/1, Product/2, Gain/1
  Product/1 -> Gain2/1
  Gain1/1 -> Add/3
  Gain2/1 -> Add/4
